simulink model "MatlabFunctionLianxi"  (Simulink 9.1)
settings: Solver=VariableStepAuto  StartTime=0.0  StopTime=10.0  RelTol=1e-3
settings Model: Creator=McQueen_Zero  LastModifiedBy=McQueen_Zero
settings DataIOCC: SaveFormat=Dataset
settings OptimizationCC: LifeSpan=auto
settings DebuggingCC: UnderspecifiedInitializationDetection=Simplified  MergeDetectMultiDrivingBlocksExec=error  SFUnexpectedBacktrackingDiag=error  SFNoUnconditionalDefaultTransitionDiag=error  SFExecutionAtInitializationDiag=warning
settings HardwareCC: ProdBitPerPointer=64  ProdBitPerSizeT=64  ProdBitPerPtrDiffT=64  ProdLargestAtomicFloat=Float  ProdIntDivRoundTo=Zero  ProdEndianess=LittleEndian  ProdWordSize=64  ProdHWDeviceType=Intel->x86-64 (Windows64)
settings ModelReferenceCC: PropagateSignalLabelsOutOfModel=on
settings CodeAppCC: StateflowObjectComments=off
settings GRTTargetCC: TargetLangStandard=C99 (ISO)  CombineOutputUpdateFcns=on  GRTInterface=off
settings ConfigComp: CovMetricSettings=dwe  CovHtmlReporting=off  CovSaveCumulativeToWorkspaceVar=off  CovSaveSingleToWorkspaceVar=off  CovExternalEMLEnable=on

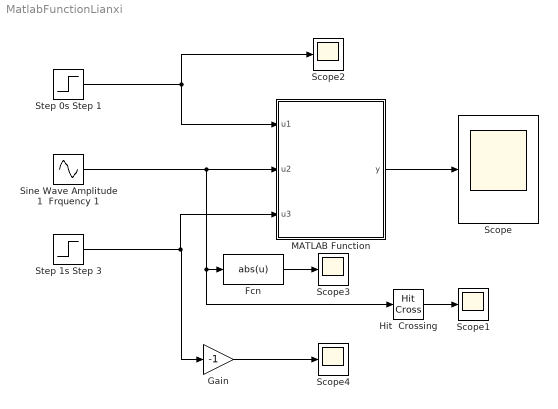
== system MatlabFunctionLianxi ==
  Fcn : Fcn  Expr=abs(u)
  Gain : Gain  Gain=-1
  Hit  Crossing : HitCross
  MATLAB Function : MATLAB Function  TreatAsAtomicUnit=on
  Scope{,1..4} (5 alike) : Scope
  Sine Wave Amplitude 1  Frquency 1 : Sin  SampleTime=0
  Step 0s Step 1 : Step  Time=0  SampleTime=0
  Step 1s Step 3 : Step  After=3  SampleTime=0
  wires:
  MATLAB Function/1(y) -> Scope/1
  Step 0s Step 1/1 -> Scope2/1, MATLAB Function/1(u1)
  Sine Wave Amplitude 1  Frquency 1/1 -> Hit  Crossing/1, Fcn/1, MATLAB Function/2(u2)
  Step 1s Step 3/1 -> MATLAB Function/3(u3), Gain/1
  Hit  Crossing/1 -> Scope1/1
  Gain/1 -> Scope4/1
  Fcn/1 -> Scope3/1

== matlab function MATLAB Function ==
  data: u1 input double; y output double; u2 input double; u3 input double
function y = mfcn(u1,u2,u3)
switch nargin
    case 1
        y = u1;
    case 2
        y = abs(u2);
    otherwise
        y = -u3;
end
end
